simulink model "bouncing_ball_2"  (R2024a)
settings: Solver=ode45  StartTime=0.0  StopTime=10  RelTol=1e-3  EnableMultiTasking=on
libraries: vrlib x2, simulink x1
settings Model: Creator=smahapat  LastModifiedBy=Miko
settings SolverCC: AlgebraicLoopSolver=TrustRegion
settings DataIOCC: LimitDataPoints=on  SaveFormat=Array  SignalLoggingSaveFormat=ModelDataLogs  ReturnWorkspaceOutputs=off
settings OptimizationCC: ExpressionDepthLimit=2147483647  LifeSpan=inf
settings DebuggingCC: UnderspecifiedInitializationDetection=Classic  MergeDetectMultiDrivingBlocksExec=none  SolverPrmCheckMsg=warning  FcnCallInpInsideContextMsg=warning  UnconnectedInputMsg=warning  UnconnectedOutputMsg=warning  UnconnectedLineMsg=warning  StateNameClashWarn=warning  SFUnexpectedBacktrackingDiag=warning  SFNoUnconditionalDefaultTransitionDiag=warning  SFExecutionAtInitializationDiag=none  ArithmeticOperatorsInVariantConditions=warning
settings HardwareCC: ProdBitPerPointer=32  ProdBitPerSizeT=32  ProdBitPerPtrDiffT=32  ProdLargestAtomicFloat=None  ProdIntDivRoundTo=Undefined  ProdEndianess=Unspecified  ProdWordSize=32  ProdHWDeviceType=32-bit Generic
settings ModelReferenceCC: PropagateSignalLabelsOutOfModel=off
settings SFSimCC: SimUseLocalCustomCode=off  SimParseCustomCode=off  CustomCodeUndefinedFunction=UseInterfaceOnly
settings RTWCC: RTWUseLocalCustomCode=off  GPUComputeCapability=3.5
settings CodeAppCC: StateflowObjectComments=on
settings GRTTargetCC: TargetLangStandard=C89/C90 (ANSI)  CombineOutputUpdateFcns=off  GRTInterface=on
settings ConfigComp: CovMetricSettings=dw  CovSaveCumulativeToWorkspaceVar=on  CovSaveSingleToWorkspaceVar=on  CovExternalEMLEnable=off

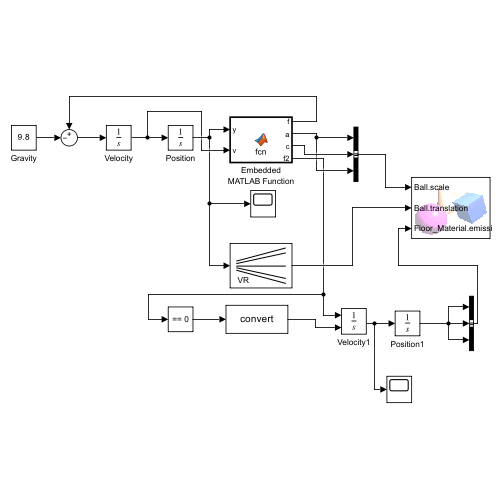
[thumbnail: Simulink's stored preview of the top-level diagram]
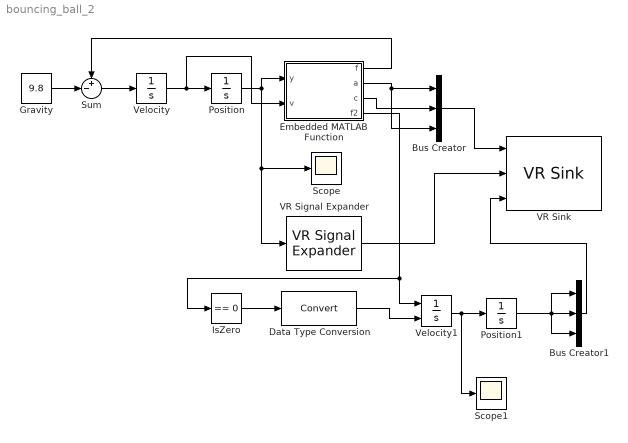
== system bouncing_ball_2 ==
  Bus Creator : BusCreator  Inputs=3
  Bus Creator1 : BusCreator  Inputs=3
  Data Type Conversion : DataTypeConversion  SaturateOnIntegerOverflow=off  RndMeth=Floor
  Embedded MATLAB Function : MATLAB Function  TreatAsAtomicUnit=on
  Gravity : Constant  Value=9.8
  IsZero : simulink/Logic and Bit Operations/Compare To Zero  relop===  OutDataTypeStr=boolean
      settings: LibrarySourceBlock=|
      | simulink/Quick Insert/Logic and Bit
      | Operations/IsZero
  Position : Integrator  InitialCondition=20
  Position1 : Integrator
  Scope : Scope
  Scope1 : Scope
  Sum : Sum  Inputs=+-|
  VR Signal Expander : vrlib/VR Signal Expander  outwidth=3  outidx=[2]
  VR Sink : vrlib/VR Sink  InstantiateOnLoad=on  SampleTime=0.01  ViewEnable=on  RemoteChange=off  RemoteView=off  FieldsWritten=Ball.scale.3.1.1.double#Ball.translation.3.1.1.double#Floor_Material.emissiveColor.3.1.1.double  WorldFileName=bouncing_ball_2.wrl  AutoView=off  VideoDimensions=[]  AllowVariableSize=off  FigureProperties=[]
  Velocity : Integrator
  Velocity1 : Integrator  ExternalReset=level hold
  wires:
  Velocity/1 -> Embedded MATLAB Function/2(v), Position/1
  Position/1 -> Embedded MATLAB Function/1(y), VR Signal Expander/1, Scope/1
  Sum/1 -> Velocity/1
  Embedded MATLAB Function/3(c) -> Bus Creator/2
  Embedded MATLAB Function/2(a) -> Bus Creator/1, Bus Creator/3
  Embedded MATLAB Function/1(f) -> Sum/1
  Gravity/1 -> Sum/2
  Bus Creator/1 -> VR Sink/1
  VR Signal Expander/1 -> VR Sink/2
  Position1/1 -> Bus Creator1/3, Bus Creator1/1, Bus Creator1/2
  Bus Creator1/1 -> VR Sink/3
  Data Type Conversion/1 -> Velocity1/2
  Embedded MATLAB Function/4(f2) -> Velocity1/1, IsZero/1
  IsZero/1 -> Data Type Conversion/1
  Velocity1/1 -> Position1/1, Scope1/1

== matlab function bouncing_ball_2/Embedded MATLAB Function ==
  data: f output; a output; c output; y input; v input; f2 output
function [f,a, c, f2] = fcn(y, v)
f2 = 0;

if y < 1e-4
    y = 1e-4;
end

if y < 1.5
    f1 = 500*(1.5-y);
    if v < 0
        f2 = -10*v;
    end
    a = sqrt(1.5^3/y);
    c = y;
else
    f1 = 0;
    a = 1.5;
    c = 1.5;
end
f = f1+f2;
